simulink model "circuitoB"  (R2021a)
settings: Solver=VariableStepAuto  StartTime=0.0  StopTime=10.0  RelTol=1e-3
model workspace (MAT data in the model file):
  Vi = 1
settings Model: Creator=phcs  LastModifiedBy=phcs

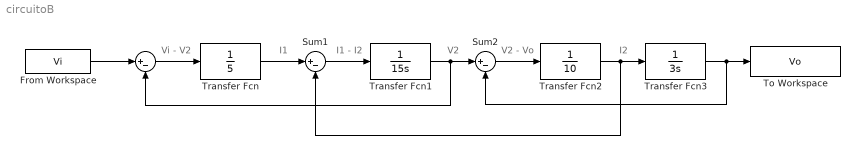
== system circuitoB ==
  note: I2
  note: V2 - Vo
  note: V2
  note: I1 - I2
  note: I1
  note: Vi - V2
  " " : Sum  Inputs=|+-
  From Workspace : FromWorkspace  VariableName=Vi
  Sum1 : Sum  Inputs=|+-
  Sum2 : Sum  Inputs=|+-
  To Workspace : ToWorkspace  VariableName=Vo  SaveFormat=Timeseries  SampleTime=-1
  Transfer Fcn : TransferFcn  Denominator=[5]
  Transfer Fcn1 : TransferFcn  Denominator=[15 0]
  Transfer Fcn2 : TransferFcn  Denominator=[10]
  Transfer Fcn3 : TransferFcn  Denominator=[3 0]
  wires:
  Transfer Fcn/1 -> Sum1/1
  Transfer Fcn1/1 -> " "/2, Sum2/1
  Sum1/1 -> Transfer Fcn1/1
  " "/1 -> Transfer Fcn/1
  From Workspace/1 -> " "/1
  Sum2/1 -> Transfer Fcn2/1
  Transfer Fcn2/1 -> Sum1/2, Transfer Fcn3/1
  Transfer Fcn3/1 -> Sum2/2, To Workspace/1
